simulink model "RT_Klausur_2011_A1_ori"  (R2013a)
settings: Solver=ode45  StartTime=0.0  StopTime=10.0  RelTol=1e-3
values from neighbouring files (symbols this model uses):
  k = 1    [RT_Klausur_SS2014.m]    (also in RT_ctrl_analyse_proc.m = 5; RT_dennis_draussen.m = 50; RT_klausurvorb.m = 0.2; RT_lab_paramLead.m)
settings Model: Creator=mainster  LastModifiedBy=mainster

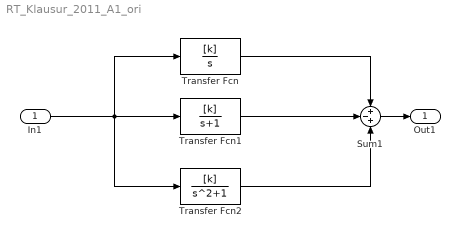
== system RT_Klausur_2011_A1_ori ==
  In1 : Inport
  Sum1 : Sum  Inputs=+-+
  Transfer Fcn : TransferFcn  Numerator=[k]  Denominator=[1 0]
  Transfer Fcn1 : TransferFcn  Numerator=[k]  Denominator=[1 1]
  Transfer Fcn2 : TransferFcn  Numerator=[k]  Denominator=[1 0 1]
  Out1 : Outport
  wires:
  In1/1 -> Transfer Fcn2/1, Transfer Fcn1/1, Transfer Fcn/1
  Sum1/1 -> Out1/1
  Transfer Fcn/1 -> Sum1/1
  Transfer Fcn1/1 -> Sum1/2
  Transfer Fcn2/1 -> Sum1/3
